simulink model "phase5_hover_control"  (R2017b)
settings: Solver=VariableStepAuto  StartTime=0.0  StopTime=10  RelTol=1e-3
values from neighbouring files (symbols this model uses):
  c = 1.140*10^-7    (= 1.14e-07)    [run_this_and_plot.m]
  k = 2.980*10^-6    (= 2.98e-06)    [run_this_and_plot.m]
  l = 0.225    [run_this_and_plot.m]
libraries: simulink x1
settings Model: Creator=chenjiasheng  LastModifiedBy=chenjiasheng

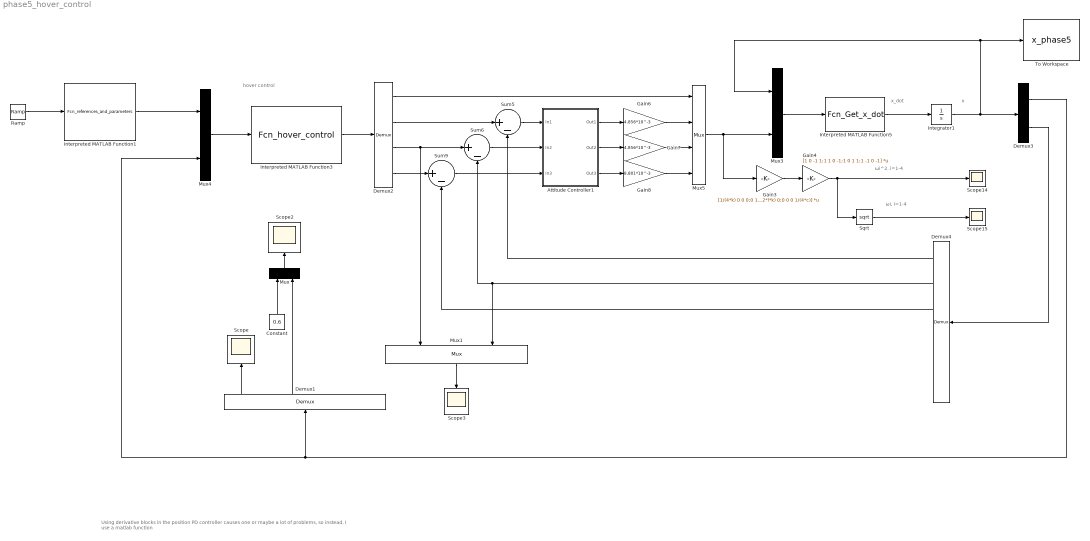
== system phase5_hover_control ==
  note: x
  note: x_dot
  note: hover control
  note: Using derivative blocks in the position PD controller causes one or maybe a lot of problems, so instead, I use a matlab function
  note: ωi, i=1-4
  note: ωi^2, i=1-4
  Attitude Controller1 : Subsystem
  Constant : Constant  Value=0.6
  Demux1 : Demux  Outputs=6
  Demux2 : Demux
  Demux3 : Demux  Outputs=2
  Demux4 : Demux  Outputs=6
  Gain3 : Gain  Gain=[1/(4*k) 0 0 0;0 1/(2*l*k) 0 0;0 0 1/(2*l*k) 0;0 0 0 1/(4*c)]  Multiplication=Matrix(K*u) (u vector)
  Gain4 : Gain  Gain=[1 0 -1 1;1 1 0 -1;1 0 1 1;1 -1 0 -1]  Multiplication=Matrix(K*u) (u vector)
  Gain6 : Gain  Gain=4.856*10^-3
  Gain7 : Gain  Gain=4.856*10^-3
  Gain8 : Gain  Gain=8.801*10^-3
  Integrator1 : Integrator  InitialCondition=x_phase4(end,:)
  Interpreted MATLAB Function1 : MATLABFcn  MATLABFcn=Fcn_references_and_parameters  OutputDimensions=15
  Interpreted MATLAB Function3 : MATLABFcn  MATLABFcn=Fcn_hover_control  OutputDimensions=4
  Interpreted MATLAB Function5 : MATLABFcn  MATLABFcn=Fcn_Get_x_dot  OutputDimensions=12
  Mux{,1,3..4} (4 alike) : Mux  Inputs=2
  Mux5 : Mux
  Ramp : simulink/Sources/Ramp  slope=1  start=0  X0=0
  Scope{,2..3,14..15} (5 alike) : Scope
  Sqrt : Sqrt  SaturateOnIntegerOverflow=on
  Sum5 : Sum  Inputs=|+-
  Sum6 : Sum  Inputs=|+-
  Sum9 : Sum  Inputs=|+-
  To Workspace : ToWorkspace  VariableName=x_phase5  SampleTime=0.01
  wires:
  Interpreted MATLAB Function1/1 -> Mux4/1
  Mux4/1 -> Interpreted MATLAB Function3/1
  Mux3/1 -> Interpreted MATLAB Function5/1
  Interpreted MATLAB Function5/1 -> Integrator1/1
  Attitude Controller1/2(Out2) -> Gain7/1
  Gain8/1 -> Mux5/4
  Demux2/4 -> Sum9/1
  Gain7/1 -> Mux5/3
  Sum6/1 -> Attitude Controller1/2(In2)
  Demux2/3 -> Sum6/1, Mux1/1
  Demux3/1 -> Demux1/1, Mux4/2
  Demux4/3 -> Sum9/2
  Sum9/1 -> Attitude Controller1/3(In3)
  Interpreted MATLAB Function3/1 -> Demux2/1
  Gain6/1 -> Mux5/2
  Attitude Controller1/3(Out3) -> Gain8/1
  Attitude Controller1/1(Out1) -> Gain6/1
  Demux3/2 -> Demux4/1
  Ramp/1 -> Interpreted MATLAB Function1/1
  Demux4/1 -> Sum5/2
  Demux4/2 -> Mux1/2, Sum6/2
  Integrator1/1 -> Mux3/1, To Workspace/1, Demux3/1
  Demux2/2 -> Sum5/1
  Mux5/1 -> Gain3/1, Mux3/2
  Sum5/1 -> Attitude Controller1/1(In1)
  Demux2/1 -> Mux5/1
  Demux1/1 -> Scope/1
  Demux1/3 -> Mux/2
  Mux/1 -> Scope2/1
  Constant/1 -> Mux/1
  Mux1/1 -> Scope3/1
  Gain4/1 -> Sqrt/1, Scope14/1
  Sqrt/1 -> Scope15/1
  Gain3/1 -> Gain4/1

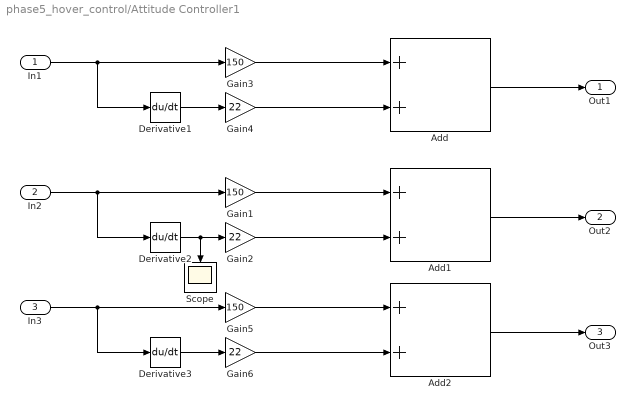
== system phase5_hover_control/Attitude Controller1 ==
  In1 : Inport
  In2 : Inport  Port=2
  In3 : Inport  Port=3
  Add : Sum
  Add1 : Sum
  Add2 : Sum
  Derivative1 : Derivative
  Derivative2 : Derivative
  Derivative3 : Derivative
  Gain1 : Gain  Gain=150
  Gain2 : Gain  Gain=22
  Gain3 : Gain  Gain=150
  Gain4 : Gain  Gain=22
  Gain5 : Gain  Gain=150
  Gain6 : Gain  Gain=22
  Scope : Scope
  Out1 : Outport
  Out2 : Outport  Port=2
  Out3 : Outport  Port=3
  wires:
  Add2/1 -> Out3/1
  Derivative3/1 -> Gain6/1
  Gain6/1 -> Add2/2
  In3/1 -> Gain5/1, Derivative3/1
  Gain5/1 -> Add2/1
  Gain1/1 -> Add1/1
  In2/1 -> Derivative2/1, Gain1/1
  Gain2/1 -> Add1/2
  Derivative2/1 -> Gain2/1, Scope/1
  Add1/1 -> Out2/1
  Add/1 -> Out1/1
  Derivative1/1 -> Gain4/1
  Gain4/1 -> Add/2
  In1/1 -> Gain3/1, Derivative1/1
  Gain3/1 -> Add/1
